simulink model "MIAC"  (R2018b)
settings: Solver=VariableStepAuto  StartTime=0.0  StopTime=50000  RelTol=1e-3
undefined symbols (not defined in the file): s
libraries: cstblocks x3, peGeneralControl x3, simulink x1, slident x1
settings Model: Creator=Trips  LastModifiedBy=Trips

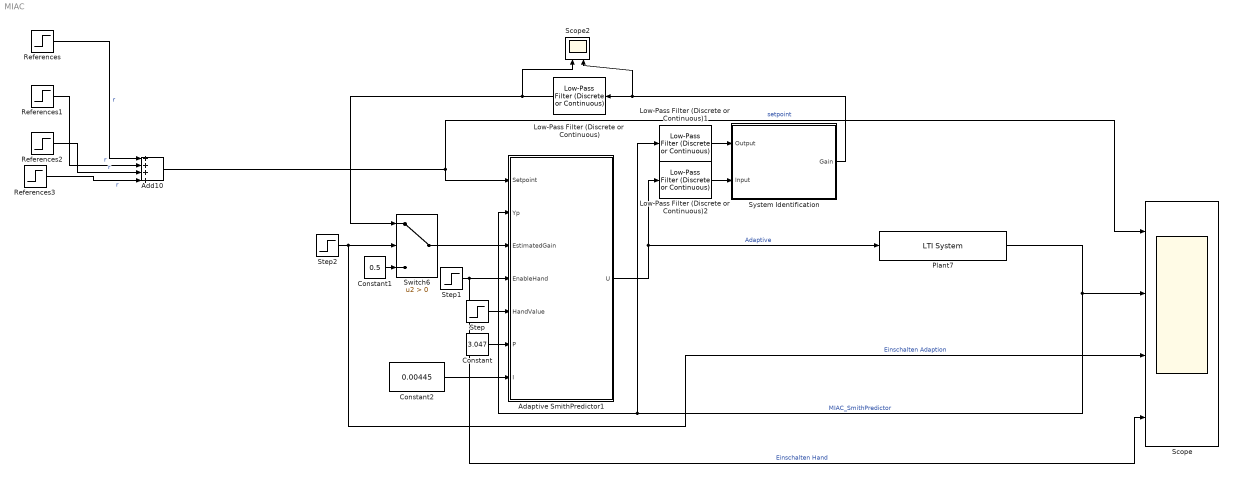
== system MIAC ==
  Adaptive SmithPredictor1 : Subsystem
  Add10 : Sum  Inputs=++++
  Constant : Constant  Value=3.047
  Constant1 : Constant  Value=0.5
  Constant2 : Constant  Value=0.00445
  Low-Pass Filter (Discrete or Continuous) : peGeneralControl/Low-Pass Filter (Discrete or Continuous)  K=1  T=1200  B=inf  A=-inf  Ts=-1
  Low-Pass Filter (Discrete or Continuous)1 : peGeneralControl/Low-Pass Filter (Discrete or Continuous)  K=1  T=1200  B=inf  A=-inf  Ts=-1
  Low-Pass Filter (Discrete or Continuous)2 : peGeneralControl/Low-Pass Filter (Discrete or Continuous)  K=1  T=1200  B=inf  A=-inf  Ts=-1
  Plant7 : cstblocks/LTI System  sys=0.5/(700*s+1)*exp(-s*600)  IC=[]
  References : Step
  References1 : Step  Time=12000  After=2
  References2 : Step  Time=18000  After=3
  References3 : Step  Time=35000  After=3
  Scope : Scope  NumInputPorts=4
  Scope2 : Scope  NumInputPorts=2
  Step : Step  Time=0  SampleTime=0
  Step1 : Step  Time=3000  Before=1  After=0  SampleTime=0
  Step2 : Step  Time=4000  SampleTime=0
  Switch6 : Switch  Criteria=u2 > Threshold
  System Identification : Subsystem
  wires:
  Low-Pass Filter (Discrete or Continuous)/1 -> Switch6/1, Scope2/1
  System Identification/1(Gain) -> Low-Pass Filter (Discrete or Continuous)/1, Scope2/2
  Plant7/1 -> Low-Pass Filter (Discrete or Continuous)1/1, Adaptive SmithPredictor1/2(Yp), Scope/2  "MIAC_SmithPredictor"
  Switch6/1 -> Adaptive SmithPredictor1/3(EstimatedGain)
  Step2/1 -> Switch6/2, Scope/3  "Einschalten Adaption"
  Low-Pass Filter (Discrete or Continuous)1/1 -> System Identification/1(Output)
  Low-Pass Filter (Discrete or Continuous)2/1 -> System Identification/2(Input)
  Adaptive SmithPredictor1/1(U) -> Low-Pass Filter (Discrete or Continuous)2/1, Plant7/1  "Adaptive"
  Constant1/1 -> Switch6/3
  References/1 -> Add10/1  "r"
  References2/1 -> Add10/3  "r"
  References3/1 -> Add10/4  "r"
  References1/1 -> Add10/2  "r"
  Add10/1 -> Scope/1, Adaptive SmithPredictor1/1(Setpoint)  "setpoint"
  Step/1 -> Adaptive SmithPredictor1/5(HandValue)
  Step1/1 -> Adaptive SmithPredictor1/4(EnableHand), Scope/4  "Einschalten Hand"
  Constant/1 -> Adaptive SmithPredictor1/6(P)
  Constant2/1 -> Adaptive SmithPredictor1/7(I)

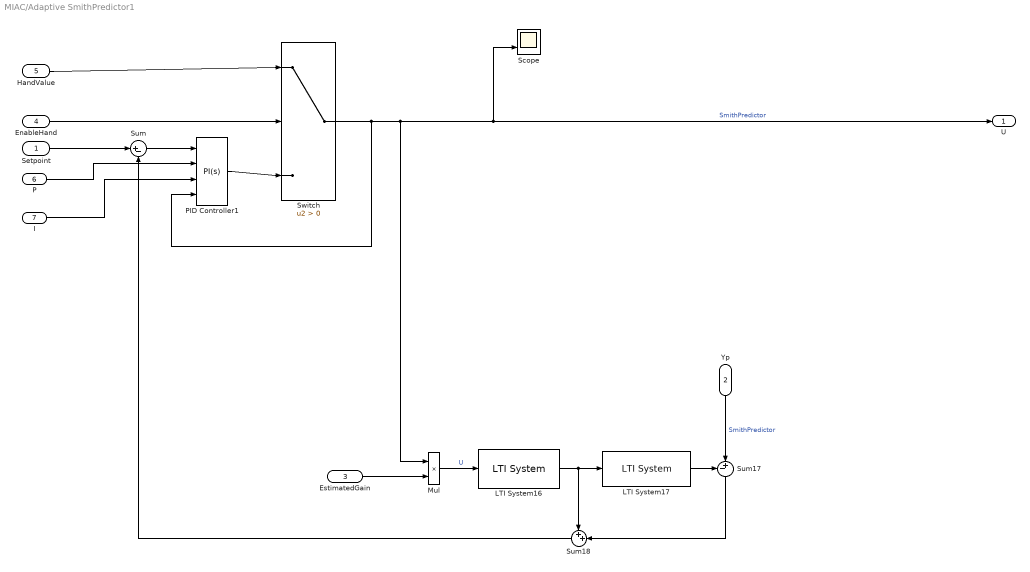
== system MIAC/Adaptive SmithPredictor1 ==
  Setpoint : Inport
  Yp : Inport  Port=2
  EstimatedGain : Inport  Port=3
  EnableHand : Inport  Port=4
  HandValue : Inport  Port=5
  P : Inport  Port=6
  I : Inport  Port=7
  LTI System16 : cstblocks/LTI System  sys=1/(700*s+1)  IC=[]
  LTI System17 : cstblocks/LTI System  sys=exp(-s*600)  IC=[]
  Mul : Product
  PID Controller1 : simulink/Continuous/PID Controller  Controller=PI  Form=Parallel  TimeDomain=Continuous-time  SampleTime=-1  IntegratorMethod=Forward Euler  FilterMethod=Forward Euler  ControllerParametersSource=external  P=3.04732259067536  I=0.00445689106465138  D=118.272348286844  UseFilter=on  N=0.00420306193364532  TunerSelectOption=Transfer Function Based (PID Tuner App)  InitialConditionSource=internal  InitialConditionForIntegrator=0  InitialConditionForFilter=0  DifferentiatorICPrevScaledInput=0  ExternalReset=none  TrackingMode=on  Kt=1  LimitOutput=on  UpperSaturationLimit=100  LowerSaturationLimit=0  LinearizeAsGain=on  AntiWindupMode=none  Kb=1  POutMin=[]  POutMax=[]  IOutMin=[]  IOutMax=[]  DOutMin=[]  DOutMax=[]  NOutMin=[]  NOutMax=[]  SumOutMin=[]  SumOutMax=[]  SaturationOutMin=[]  SaturationOutMax=[]  PParamMin=[]  PParamMax=[]  IParamMin=[]  IParamMax=[]  DParamMin=[]  DParamMax=[]  NParamMin=[]  NParamMax=[]  KbParamMin=[]  KbParamMax=[]  KtParamMin=[]  KtParamMax=[]  KbOutMin=[]  KbOutMax=[]  KtOutMin=[]  KtOutMax=[]  IntegratorOutMin=[]  IntegratorOutMax=[]  FilterOutMin=[]  FilterOutMax=[]  SumI1OutMin=[]  SumI1OutMax=[]  SumI2OutMin=[]  SumI2OutMax=[]  SumI3OutMin=[]  SumI3OutMax=[]  SumI4OutMin=[]  SumI4OutMax=[]  SumDOutMin=[]  SumDOutMax=[]  DifferentiatorOutMin=[]  DifferentiatorOutMax=[]  FilterDiffOutCoefMin=[]  FilterDiffOutCoefMax=[]  ReciprocalOutMin=[]  ReciprocalOutMax=[]  SumDenOutMin=[]  SumDenOutMax=[]  SumNumOutMin=[]  SumNumOutMax=[]  DivideOutMin=[]  DivideOutMax=[]  IntegratorContinuousStateAttributes=''  IntegratorStateMustResolveToSignalObject=off  IntegratorRTWStateStorageClass=Auto  FilterContinuousStateAttributes=''  FilterStateMustResolveToSignalObject=off  FilterRTWStateStorageClass=Auto  ParallelPVariant=ExternalParameters  IdealPVariant=Disabled  IVariant=ExternalParameters  DVariant=Disabled  IntegratorVariant=Continuous  SatVariant=Enabled  AWVariant=Passthrough  PCopyVariant=Disabled  TRVariant=Enabled  FdbkBlocksVariant=Forward  IdealPFdbkVariant=Disabled  SatFdbkVariant=Disabled  DerivativeFilterVariant=Disabled  NVariant=Disabled  NCopyVariant=Disabled_SignalSpec  FilterICVariant=Disabled  IntegratorICVariant=InternalICs  ExternalResetVariant=Disabled  TRSumVariant=TrackingMode  SumFdbkVariant=Disabled  SumVariant=Sum_PI
  Scope : Scope  NumInputPorts=2
  Sum : Sum  Inputs=|+-
  Sum17 : Sum  Inputs=-+|
  Sum18 : Sum  Inputs=++|
  Switch : Switch  Criteria=u2 > Threshold
  U : Outport
  wires:
  Setpoint/1 -> Sum/1
  Sum/1 -> PID Controller1/1
  Switch/1 -> PID Controller1/4, Mul/1, U/1, Scope/2  "SmithPredictor"
  Yp/1 -> Sum17/2  "SmithPredictor"
  LTI System16/1 -> LTI System17/1, Sum18/1
  Sum18/1 -> Sum/2
  LTI System17/1 -> Sum17/1
  Sum17/1 -> Sum18/2
  Mul/1 -> LTI System16/1  "U"
  EstimatedGain/1 -> Mul/2
  PID Controller1/1 -> Switch/3
  HandValue/1 -> Switch/1
  EnableHand/1 -> Switch/2
  P/1 -> PID Controller1/2
  I/1 -> PID Controller1/3

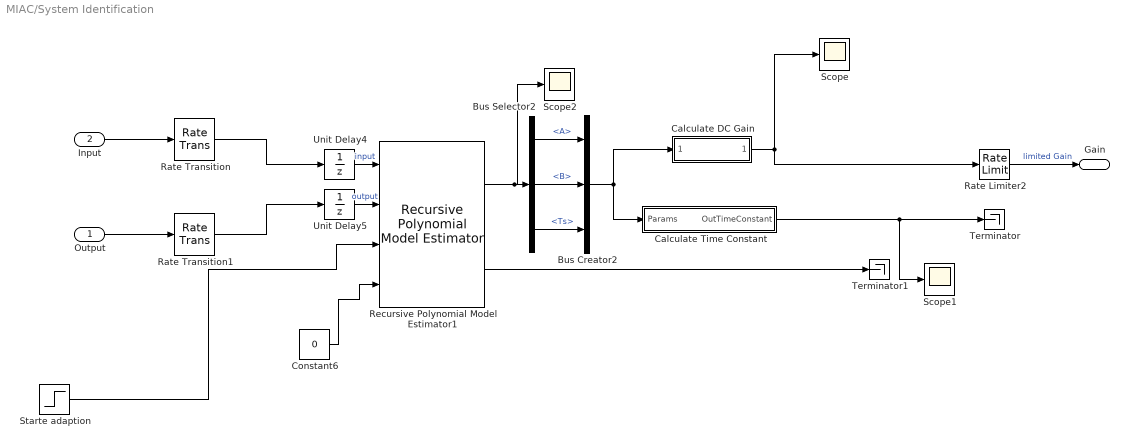
== system MIAC/System Identification ==
  Output : Inport
  Input : Inport  Port=2
  Bus Creator2 : BusCreator  Inputs=3
  Bus Selector2 : BusSelector  OutputSignals=A,B,Ts
  Calculate DC Gain : Subsystem
  Calculate Time Constant : Subsystem
  Constant6 : Constant  Value=0  SampleTime=1
  Rate Limiter2 : RateLimiter  SampleTimeMode=inherited
  Rate Transition : RateTransition  OutPortSampleTime=1
  Rate Transition1 : RateTransition  OutPortSampleTime=1
  Recursive Polynomial Model Estimator1 : slident/Estimators/Recursive Polynomial Model Estimator  ModelStructure=ARX  InitialEstimateSource=None  A0=1  B0=1  C0=1  D0=1  F0=1  nk=1  P0=1  InitialInputs=0  InitialOutputs=0  History=Infinite  WindowLength=2000  EstimationMethod=Forgetting Factor  AdaptationParameter=1  HasTimeVaryingAdaptationParameter=off  NormalizationBias=eps  OutputError=on  OutputP=off  AddEnablePort=on  ExternalReset=Rising  InputProcessing=Sample-based  Ts=1
      settings: SourceProductName=System Identification Toolbox  SourceProductBaseCode=ID
  Scope : Scope
  Scope1 : Scope
  Scope2 : Scope
  Starte adaption : Step  Time=0  SampleTime=1
  Terminator : Terminator
  Terminator1 : Terminator
  Unit Delay4 : UnitDelay  InitialCondition=[0]
  Unit Delay5 : UnitDelay
  Gain : Outport
  wires:
  Bus Selector2/1 -> Bus Creator2/1  "<A>"
  Recursive Polynomial Model Estimator1/1 -> Scope2/1, Bus Selector2/1
  Bus Selector2/3 -> Bus Creator2/3  "<Ts>"
  Bus Selector2/2 -> Bus Creator2/2  "<B>"
  Bus Creator2/1 -> Calculate DC Gain/1(Params), Calculate Time Constant/1(Params)
  Recursive Polynomial Model Estimator1/2 -> Terminator1/1
  Rate Limiter2/1 -> Gain/1  "limited Gain"
  Calculate Time Constant/1("OutTimeConstant ") -> Scope1/1, Terminator/1
  Constant6/1 -> Recursive Polynomial Model Estimator1/4
  Unit Delay4/1 -> Recursive Polynomial Model Estimator1/1  "input"
  Unit Delay5/1 -> Recursive Polynomial Model Estimator1/2  "output"
  Input/1 -> Rate Transition/1
  Output/1 -> Rate Transition1/1
  Rate Transition/1 -> Unit Delay4/1
  Rate Transition1/1 -> Unit Delay5/1
  Starte adaption/1 -> Recursive Polynomial Model Estimator1/3
  Calculate DC Gain/1(DCGain) -> Rate Limiter2/1, Scope/1

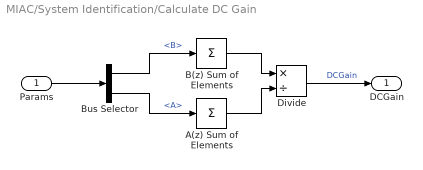
== system MIAC/System Identification/Calculate DC Gain ==
  Params : Inport
  A(z) Sum of Elements : Sum  Inputs=+
  B(z) Sum of Elements : Sum  Inputs=+
  Bus Selector : BusSelector  OutputSignals=B,A
  Divide : Product  Inputs=*/
  DCGain : Outport
  wires:
  A(z) Sum of Elements/1 -> Divide/2
  B(z) Sum of Elements/1 -> Divide/1
  Params/1 -> Bus Selector/1
  Bus Selector/1 -> B(z) Sum of Elements/1  "<B>"
  Bus Selector/2 -> A(z) Sum of Elements/1  "<A>"
  Divide/1 -> DCGain/1  "DCGain"

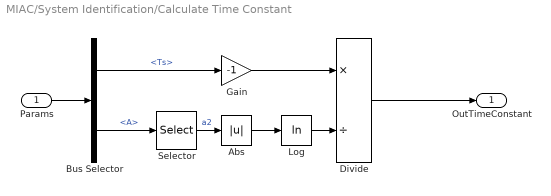
== system MIAC/System Identification/Calculate Time Constant ==
  Params : Inport
  Abs : Abs
  Bus Selector : BusSelector  OutputSignals=Ts,A
  Divide : Product  Inputs=*/
  Gain : Gain  Gain=-1
  Log : Math  Operator=log  SaturateOnIntegerOverflow=on
  Selector : Selector  InputPortWidth=2  IndexOptions=Starting index (dialog)  Indices=[2]  OutputSizes=1
  "OutTimeConstant " : Outport
  wires:
  Params/1 -> Bus Selector/1
  Bus Selector/1 -> Gain/1  "<Ts>"
  Bus Selector/2 -> Selector/1  "<A>"
  Selector/1 -> Abs/1  "a2"
  Gain/1 -> Divide/1
  Log/1 -> Divide/2
  Divide/1 -> "OutTimeConstant "/1
  Abs/1 -> Log/1
